simulink library "DEM_lib"  (Simulink 7.4)
settings: Solver=FixedStepDiscrete  StartTime=0.0  StopTime=Inf  FixedStep=0.001  RelTol=1e-3
undefined symbols (not defined in the file or in its folder): BCU_Drive_St, BCU_FastCharge_St, BCU_SlowCharge_St, COR_Fault_Bus, CTC_DefaultOffline_CtrCmd, CTC_DriveEmgyDcnct_CtrCmd, CTC_DriveOffline_CtrCmd, CTC_DriveOnline_CtrCmd, EHP_Fault_Bus, FCM_Fault_Bus, SCM_Fault_Bus
libraries: Defined_Functionality x82, simulink x2
(part 3 of 4)

== system DEM_lib/Diagnostic_Event_Management/fault_collect/BTM_Fault_Confirmed/Subsystem1 ==
  ifault : Inport  OutDataType=fixdt(1, 16)  OutScaling=2^0
  Terminator : Terminator
  Terminator1 : Terminator
  Terminator2 : Terminator
  diagnostic1 : Defined_Functionality/diagnostic1  SystemSampleTime=-1  afl_inc=DEMc_MdlTempOverfault_inc  afl_dec=DEMc_MdlTempOverfault_dec  afl_threshold=DEMc_MdlTempOverfault_AflThrld  aff_threshold=DEMc_MdlTempOverfault_AffThrld
      settings: AttributesFormatString=[AFL_INCREMENT=%<afl_inc>]\n[AFL_DECREMENT=%<afl_dec>]\n[AFL_THRESHOLD=%<afl_threshold>]\n[AFF_THRESHOLD=%<aff_threshold>]
  cfault : Outport  OutDataType=fixdt(1, 16)  OutScaling=2^0
  wires:
  ifault/1 -> diagnostic1/1
  diagnostic1/2 -> cfault/1
  diagnostic1/1 -> Terminator/1
  diagnostic1/4 -> Terminator1/1
  diagnostic1/3 -> Terminator2/1

== system DEM_lib/Diagnostic_Event_Management/fault_collect/BTM_Fault_Confirmed/Subsystem2 ==
  ifault : Inport  OutDataType=fixdt(1, 16)  OutScaling=2^0
  Terminator : Terminator
  Terminator1 : Terminator
  Terminator2 : Terminator
  diagnostic1 : Defined_Functionality/diagnostic1  SystemSampleTime=-1  afl_inc=DEMc_MdlTempOverwarn_inc  afl_dec=DEMc_MdlTempOverwarn_dec  afl_threshold=DEMc_MdlTempOverwarn_AflThrld  aff_threshold=DEMc_MdlTempOverwarn_AffThrld
      settings: AttributesFormatString=[AFL_INCREMENT=%<afl_inc>]\n[AFL_DECREMENT=%<afl_dec>]\n[AFL_THRESHOLD=%<afl_threshold>]\n[AFF_THRESHOLD=%<aff_threshold>]
  cfault : Outport  OutDataType=fixdt(1, 16)  OutScaling=2^0
  wires:
  diagnostic1/3 -> Terminator2/1
  diagnostic1/4 -> Terminator1/1
  diagnostic1/1 -> Terminator/1
  diagnostic1/2 -> cfault/1
  ifault/1 -> diagnostic1/1

== system DEM_lib/Diagnostic_Event_Management/fault_collect/BTM_Fault_Confirmed/Subsystem3 ==
  ifault : Inport  OutDataType=fixdt(1, 16)  OutScaling=2^0
  Terminator : Terminator
  Terminator1 : Terminator
  Terminator2 : Terminator
  diagnostic1 : Defined_Functionality/diagnostic1  SystemSampleTime=-1  afl_inc=DEMc_MdlTempUnderwarn_inc  afl_dec=DEMc_MdlTempUnderwarn_dec  afl_threshold=DEMc_MdlTempUnderwarn_AflThrld  aff_threshold=DEMc_MdlTempUnderwarn_AffThrld
      settings: AttributesFormatString=[AFL_INCREMENT=%<afl_inc>]\n[AFL_DECREMENT=%<afl_dec>]\n[AFL_THRESHOLD=%<afl_threshold>]\n[AFF_THRESHOLD=%<aff_threshold>]
  cfault : Outport  OutDataType=fixdt(1, 16)  OutScaling=2^0
  wires:
  diagnostic1/3 -> Terminator2/1
  diagnostic1/4 -> Terminator1/1
  diagnostic1/1 -> Terminator/1
  diagnostic1/2 -> cfault/1
  ifault/1 -> diagnostic1/1

== system DEM_lib/Diagnostic_Event_Management/fault_collect/BTM_Fault_Confirmed/Subsystem4 ==
  ifault : Inport  OutDataType=fixdt(1, 16)  OutScaling=2^0
  Terminator : Terminator
  Terminator1 : Terminator
  Terminator2 : Terminator
  diagnostic1 : Defined_Functionality/diagnostic1  SystemSampleTime=-1  afl_inc=DEMc_MdlTempDifOverwarn_inc  afl_dec=DEMc_MdlTempDifOverwarn_dec  afl_threshold=DEMc_MdlTempDifOverwarn_AflThrld  aff_threshold=DEMc_MdlTempDifOverwarn_AffThrld
      settings: AttributesFormatString=[AFL_INCREMENT=%<afl_inc>]\n[AFL_DECREMENT=%<afl_dec>]\n[AFL_THRESHOLD=%<afl_threshold>]\n[AFF_THRESHOLD=%<aff_threshold>]
  cfault : Outport  OutDataType=fixdt(1, 16)  OutScaling=2^0
  wires:
  ifault/1 -> diagnostic1/1
  diagnostic1/2 -> cfault/1
  diagnostic1/1 -> Terminator/1
  diagnostic1/4 -> Terminator1/1
  diagnostic1/3 -> Terminator2/1

== system DEM_lib/Diagnostic_Event_Management/fault_collect/BTM_Fault_Confirmed/Subsystem5 ==
  ifault : Inport  OutDataType=fixdt(1, 16)  OutScaling=2^0
  Terminator : Terminator
  Terminator1 : Terminator
  Terminator2 : Terminator
  diagnostic1 : Defined_Functionality/diagnostic1  SystemSampleTime=-1  afl_inc=DEMc_MdlTempDifOverfault_inc  afl_dec=DEMc_MdlTempDifOverfault_dec  afl_threshold=DEMc_MdlTempDifOverfault_AflThrld  aff_threshold=DEMc_MdlTempDifOverfault_AffThrld
      settings: AttributesFormatString=[AFL_INCREMENT=%<afl_inc>]\n[AFL_DECREMENT=%<afl_dec>]\n[AFL_THRESHOLD=%<afl_threshold>]\n[AFF_THRESHOLD=%<aff_threshold>]
  cfault : Outport  OutDataType=fixdt(1, 16)  OutScaling=2^0
  wires:
  diagnostic1/3 -> Terminator2/1
  diagnostic1/4 -> Terminator1/1
  diagnostic1/1 -> Terminator/1
  diagnostic1/2 -> cfault/1
  ifault/1 -> diagnostic1/1

== system DEM_lib/Diagnostic_Event_Management/fault_collect/BTM_Fault_Confirmed/Subsystem6 ==
  ifault : Inport  OutDataType=fixdt(1, 16)  OutScaling=2^0
  Terminator : Terminator
  Terminator1 : Terminator
  Terminator2 : Terminator
  diagnostic1 : Defined_Functionality/diagnostic1  SystemSampleTime=-1  afl_inc=DEMc_MdlTempOverfatal_inc  afl_dec=DEMc_MdlTempOverfatal_dec  afl_threshold=DEMc_MdlTempOverfatal_AflThrld  aff_threshold=DEMc_MdlTempOverfatal_AffThrld
      settings: AttributesFormatString=[AFL_INCREMENT=%<afl_inc>]\n[AFL_DECREMENT=%<afl_dec>]\n[AFL_THRESHOLD=%<afl_threshold>]\n[AFF_THRESHOLD=%<aff_threshold>]
  cfault : Outport  OutDataType=fixdt(1, 16)  OutScaling=2^0
  wires:
  diagnostic1/3 -> Terminator2/1
  diagnostic1/4 -> Terminator1/1
  diagnostic1/1 -> Terminator/1
  diagnostic1/2 -> cfault/1
  ifault/1 -> diagnostic1/1

== system DEM_lib/Diagnostic_Event_Management/fault_collect/BTM_Fault_Confirmed/Subsystem7 ==
  ifault : Inport  OutDataType=fixdt(1, 16)  OutScaling=2^0
  Terminator : Terminator
  Terminator1 : Terminator
  Terminator2 : Terminator
  diagnostic1 : Defined_Functionality/diagnostic1  SystemSampleTime=-1  afl_inc=DEMc_BMUMaxTempOverwarn_inc  afl_dec=DEMc_BMUMaxTempOverwarn_dec  afl_threshold=DEMc_BMUMaxTempOverwarn_AflThrld  aff_threshold=DEMc_BMUMaxTempOverwarn_AffThrld
      settings: AttributesFormatString=[AFL_INCREMENT=%<afl_inc>]\n[AFL_DECREMENT=%<afl_dec>]\n[AFL_THRESHOLD=%<afl_threshold>]\n[AFF_THRESHOLD=%<aff_threshold>]
  cfault : Outport  OutDataType=fixdt(1, 16)  OutScaling=2^0
  wires:
  ifault/1 -> diagnostic1/1
  diagnostic1/2 -> cfault/1
  diagnostic1/1 -> Terminator/1
  diagnostic1/4 -> Terminator1/1
  diagnostic1/3 -> Terminator2/1

== system DEM_lib/Diagnostic_Event_Management/fault_collect/BTM_Fault_Confirmed/Subsystem8 ==
  ifault : Inport  OutDataType=fixdt(1, 16)  OutScaling=2^0
  Terminator : Terminator
  Terminator1 : Terminator
  Terminator2 : Terminator
  diagnostic1 : Defined_Functionality/diagnostic1  SystemSampleTime=-1  afl_inc=DEMc_BCUMaxTempOverwarn_inc  afl_dec=DEMc_BCUMaxTempOverwarn_dec  afl_threshold=DEMc_BCUMaxTempOverwarn_AflThrld  aff_threshold=DEMc_BCUMaxTempOverwarn_AffThrld
      settings: AttributesFormatString=[AFL_INCREMENT=%<afl_inc>]\n[AFL_DECREMENT=%<afl_dec>]\n[AFL_THRESHOLD=%<afl_threshold>]\n[AFF_THRESHOLD=%<aff_threshold>]
  cfault : Outport  OutDataType=fixdt(1, 16)  OutScaling=2^0
  wires:
  diagnostic1/3 -> Terminator2/1
  diagnostic1/4 -> Terminator1/1
  diagnostic1/1 -> Terminator/1
  diagnostic1/2 -> cfault/1
  ifault/1 -> diagnostic1/1

== system DEM_lib/Diagnostic_Event_Management/fault_collect/COR_Fault_Confirmed/Subsystem1 ==
  ifault : Inport  OutDataType=fixdt(1, 16)  OutScaling=2^0
  Terminator : Terminator
  Terminator1 : Terminator
  Terminator2 : Terminator
  diagnostic1 : Defined_Functionality/diagnostic1  SystemSampleTime=-1  afl_inc=DEMc_CellCDcsefault_inc  afl_dec=DEMc_CellCDcsefault_dec  afl_threshold=DEMc_CellCDcsefault_AflThrld  aff_threshold=DEMc_CellCDcsefault_AffThrld
      settings: AttributesFormatString=[AFL_INCREMENT=%<afl_inc>]\n[AFL_DECREMENT=%<afl_dec>]\n[AFL_THRESHOLD=%<afl_threshold>]\n[AFF_THRESHOLD=%<aff_threshold>]
  cfault : Outport  OutDataType=fixdt(1, 16)  OutScaling=2^0
  wires:
  ifault/1 -> diagnostic1/1
  diagnostic1/2 -> cfault/1
  diagnostic1/1 -> Terminator/1
  diagnostic1/4 -> Terminator1/1
  diagnostic1/3 -> Terminator2/1

== system DEM_lib/Diagnostic_Event_Management/fault_collect/COR_Fault_Confirmed/Subsystem5 ==
  ifault : Inport  OutDataType=fixdt(1, 16)  OutScaling=2^0
  Terminator : Terminator
  Terminator1 : Terminator
  Terminator2 : Terminator
  diagnostic1 : Defined_Functionality/diagnostic1  SystemSampleTime=-1  afl_inc=DEMc_CellRDcsefault_inc  afl_dec=DEMc_CellRDcsefault_dec  afl_threshold=DEMc_CellRDcsefault_AflThrld  aff_threshold=DEMc_CellRDcsefault_AffThrld
      settings: AttributesFormatString=[AFL_INCREMENT=%<afl_inc>]\n[AFL_DECREMENT=%<afl_dec>]\n[AFL_THRESHOLD=%<afl_threshold>]\n[AFF_THRESHOLD=%<aff_threshold>]
  cfault : Outport  OutDataType=fixdt(1, 16)  OutScaling=2^0
  wires:
  diagnostic1/3 -> Terminator2/1
  diagnostic1/4 -> Terminator1/1
  diagnostic1/1 -> Terminator/1
  diagnostic1/2 -> cfault/1
  ifault/1 -> diagnostic1/1

== system DEM_lib/Diagnostic_Event_Management/fault_collect/COR_Fault_Confirmed/Subsystem8 ==
  ifault : Inport  OutDataType=fixdt(1, 16)  OutScaling=2^0
  Terminator : Terminator
  Terminator1 : Terminator
  Terminator2 : Terminator
  diagnostic1 : Defined_Functionality/diagnostic1  SystemSampleTime=-1  afl_inc=DEMc_CellRIcsefault_inc  afl_dec=DEMc_CellRIcsefault_dec  afl_threshold=DEMc_CellRIcsefault_AflThrld  aff_threshold=DEMc_CellRIcsefault_AffThrld
      settings: AttributesFormatString=[AFL_INCREMENT=%<afl_inc>]\n[AFL_DECREMENT=%<afl_dec>]\n[AFL_THRESHOLD=%<afl_threshold>]\n[AFF_THRESHOLD=%<aff_threshold>]
  cfault : Outport  OutDataType=fixdt(1, 16)  OutScaling=2^0
  wires:
  ifault/1 -> diagnostic1/1
  diagnostic1/2 -> cfault/1
  diagnostic1/1 -> Terminator/1
  diagnostic1/4 -> Terminator1/1
  diagnostic1/3 -> Terminator2/1

== system DEM_lib/Diagnostic_Event_Management/fault_collect/CTC_Fault_Confirmed/Subsystem1 ==
  ifault : Inport  OutDataType=fixdt(1, 16)  OutScaling=2^0
  Terminator : Terminator
  Terminator1 : Terminator
  Terminator2 : Terminator
  diagnostic1 : Defined_Functionality/diagnostic1  SystemSampleTime=-1  afl_inc=DEMc_PosCtrStuckOpenfault_inc  afl_dec=DEMc_PosCtrStuckOpenfault_dec  afl_threshold=DEMc_PosCtrStuckOpenfault_AflThrld  aff_threshold=DEMc_PosCtrStuckOpenfault_AffThrld
      settings: AttributesFormatString=[AFL_INCREMENT=%<afl_inc>]\n[AFL_DECREMENT=%<afl_dec>]\n[AFL_THRESHOLD=%<afl_threshold>]\n[AFF_THRESHOLD=%<aff_threshold>]
  cfault : Outport  OutDataType=fixdt(1, 16)  OutScaling=2^0
  wires:
  ifault/1 -> diagnostic1/1
  diagnostic1/2 -> cfault/1
  diagnostic1/1 -> Terminator/1
  diagnostic1/4 -> Terminator1/1
  diagnostic1/3 -> Terminator2/1

== system DEM_lib/Diagnostic_Event_Management/fault_collect/CTC_Fault_Confirmed/Subsystem10 ==
  ifault : Inport  OutDataType=fixdt(1, 16)  OutScaling=2^0
  Terminator : Terminator
  Terminator1 : Terminator
  Terminator2 : Terminator
  diagnostic1 : Defined_Functionality/diagnostic1  SystemSampleTime=-1  afl_inc=DEMc_HVEmcyDcnctTmOverfault_inc  afl_dec=DEMc_HVEmcyDcnctTmOverfault_dec  afl_threshold=DEMc_HVEmcyDcnctTmOverfault_AflThrld  aff_threshold=DEMc_HVEmcyDcnctTmOverfault_AffThrld
      settings: AttributesFormatString=[AFL_INCREMENT=%<afl_inc>]\n[AFL_DECREMENT=%<afl_dec>]\n[AFL_THRESHOLD=%<afl_threshold>]\n[AFF_THRESHOLD=%<aff_threshold>]
  cfault : Outport  OutDataType=fixdt(1, 16)  OutScaling=2^0
  wires:
  ifault/1 -> diagnostic1/1
  diagnostic1/2 -> cfault/1
  diagnostic1/1 -> Terminator/1
  diagnostic1/4 -> Terminator1/1
  diagnostic1/3 -> Terminator2/1

== system DEM_lib/Diagnostic_Event_Management/fault_collect/CTC_Fault_Confirmed/Subsystem11 ==
  ifault : Inport  OutDataType=fixdt(1, 16)  OutScaling=2^0
  Terminator : Terminator
  Terminator1 : Terminator
  Terminator2 : Terminator
  diagnostic1 : Defined_Functionality/diagnostic1  SystemSampleTime=-1  afl_inc=DEMc_PrecCurOverfault_inc  afl_dec=DEMc_PrecCurOverfault_dec  afl_threshold=DEMc_PrecCurOverfault_AflThrld  aff_threshold=DEMc_PrecCurOverfault_AffThrld
      settings: AttributesFormatString=[AFL_INCREMENT=%<afl_inc>]\n[AFL_DECREMENT=%<afl_dec>]\n[AFL_THRESHOLD=%<afl_threshold>]\n[AFF_THRESHOLD=%<aff_threshold>]
  cfault : Outport  OutDataType=fixdt(1, 16)  OutScaling=2^0
  wires:
  diagnostic1/3 -> Terminator2/1
  diagnostic1/4 -> Terminator1/1
  diagnostic1/1 -> Terminator/1
  diagnostic1/2 -> cfault/1
  ifault/1 -> diagnostic1/1

== system DEM_lib/Diagnostic_Event_Management/fault_collect/CTC_Fault_Confirmed/Subsystem12 ==
  ifault : Inport  OutDataType=fixdt(1, 16)  OutScaling=2^0
  Terminator : Terminator
  Terminator1 : Terminator
  Terminator2 : Terminator
  diagnostic1 : Defined_Functionality/diagnostic1  SystemSampleTime=-1  afl_inc=DEMc_HVCnctCurOverfault_inc  afl_dec=DEMc_HVCnctCurOverfault_dec  afl_threshold=DEMc_HVCnctCurOverfault_AflThrld  aff_threshold=DEMc_HVCnctCurOverfault_AffThrld
      settings: AttributesFormatString=[AFL_INCREMENT=%<afl_inc>]\n[AFL_DECREMENT=%<afl_dec>]\n[AFL_THRESHOLD=%<afl_threshold>]\n[AFF_THRESHOLD=%<aff_threshold>]
  cfault : Outport  OutDataType=fixdt(1, 16)  OutScaling=2^0
  wires:
  ifault/1 -> diagnostic1/1
  diagnostic1/2 -> cfault/1
  diagnostic1/1 -> Terminator/1
  diagnostic1/4 -> Terminator1/1
  diagnostic1/3 -> Terminator2/1

== system DEM_lib/Diagnostic_Event_Management/fault_collect/CTC_Fault_Confirmed/Subsystem3 ==
  ifault : Inport  OutDataType=fixdt(1, 16)  OutScaling=2^0
  Terminator : Terminator
  Terminator1 : Terminator
  Terminator2 : Terminator
  diagnostic1 : Defined_Functionality/diagnostic1  SystemSampleTime=-1  afl_inc=DEMc_PosCtrStuckCldfault_inc  afl_dec=DEMc_PosCtrStuckCldfault_dec  afl_threshold=DEMc_PosCtrStuckCldfault_AflThrld  aff_threshold=DEMc_PosCtrStuckCldfault_AffThrld
      settings: AttributesFormatString=[AFL_INCREMENT=%<afl_inc>]\n[AFL_DECREMENT=%<afl_dec>]\n[AFL_THRESHOLD=%<afl_threshold>]\n[AFF_THRESHOLD=%<aff_threshold>]
  cfault : Outport  OutDataType=fixdt(1, 16)  OutScaling=2^0
  wires:
  diagnostic1/3 -> Terminator2/1
  diagnostic1/4 -> Terminator1/1
  diagnostic1/1 -> Terminator/1
  diagnostic1/2 -> cfault/1
  ifault/1 -> diagnostic1/1

== system DEM_lib/Diagnostic_Event_Management/fault_collect/CTC_Fault_Confirmed/Subsystem4 ==
  ifault : Inport  OutDataType=fixdt(1, 16)  OutScaling=2^0
  Terminator : Terminator
  Terminator1 : Terminator
  Terminator2 : Terminator
  diagnostic1 : Defined_Functionality/diagnostic1  SystemSampleTime=-1  afl_inc=DEMc_NegCtrtStuckOpenfault_inc  afl_dec=DEMc_NegCtrtStuckOpenfault_dec  afl_threshold=DEMc_NegCtrtStuckOpenfault_AflThrld  aff_threshold=DEMc_NegCtrtStuckOpenfault_AffThrld
      settings: AttributesFormatString=[AFL_INCREMENT=%<afl_inc>]\n[AFL_DECREMENT=%<afl_dec>]\n[AFL_THRESHOLD=%<afl_threshold>]\n[AFF_THRESHOLD=%<aff_threshold>]
  cfault : Outport  OutDataType=fixdt(1, 16)  OutScaling=2^0
  wires:
  ifault/1 -> diagnostic1/1
  diagnostic1/2 -> cfault/1
  diagnostic1/1 -> Terminator/1
  diagnostic1/4 -> Terminator1/1
  diagnostic1/3 -> Terminator2/1

== system DEM_lib/Diagnostic_Event_Management/fault_collect/CTC_Fault_Confirmed/Subsystem5 ==
  ifault : Inport  OutDataType=fixdt(1, 16)  OutScaling=2^0
  Terminator : Terminator
  Terminator1 : Terminator
  Terminator2 : Terminator
  diagnostic1 : Defined_Functionality/diagnostic1  SystemSampleTime=-1  afl_inc=DEMc_NegCtrStuckCldfault_inc  afl_dec=DEMc_NegCtrStuckCldfault_dec  afl_threshold=DEMc_NegCtrStuckCldfault_AflThrld  aff_threshold=DEMc_NegCtrStuckCldfault_AffThrld
      settings: AttributesFormatString=[AFL_INCREMENT=%<afl_inc>]\n[AFL_DECREMENT=%<afl_dec>]\n[AFL_THRESHOLD=%<afl_threshold>]\n[AFF_THRESHOLD=%<aff_threshold>]
  cfault : Outport  OutDataType=fixdt(1, 16)  OutScaling=2^0
  wires:
  diagnostic1/3 -> Terminator2/1
  diagnostic1/4 -> Terminator1/1
  diagnostic1/1 -> Terminator/1
  diagnostic1/2 -> cfault/1
  ifault/1 -> diagnostic1/1

== system DEM_lib/Diagnostic_Event_Management/fault_collect/CTC_Fault_Confirmed/Subsystem6 ==
  ifault : Inport  OutDataType=fixdt(1, 16)  OutScaling=2^0
  Terminator : Terminator
  Terminator1 : Terminator
  Terminator2 : Terminator
  diagnostic1 : Defined_Functionality/diagnostic1  SystemSampleTime=-1  afl_inc=DEMc_PrecTmOverfault_inc  afl_dec=DEMc_PrecTmOverfault_dec  afl_threshold=DEMc_PrecTmOverfault_AflThrld  aff_threshold=DEMc_PrecTmOverfault_AffThrld
      settings: AttributesFormatString=[AFL_INCREMENT=%<afl_inc>]\n[AFL_DECREMENT=%<afl_dec>]\n[AFL_THRESHOLD=%<afl_threshold>]\n[AFF_THRESHOLD=%<aff_threshold>]
  cfault : Outport  OutDataType=fixdt(1, 16)  OutScaling=2^0
  wires:
  ifault/1 -> diagnostic1/1
  diagnostic1/2 -> cfault/1
  diagnostic1/1 -> Terminator/1
  diagnostic1/4 -> Terminator1/1
  diagnostic1/3 -> Terminator2/1

== system DEM_lib/Diagnostic_Event_Management/fault_collect/CTC_Fault_Confirmed/Subsystem7 ==
  ifault : Inport  OutDataType=fixdt(1, 16)  OutScaling=2^0
  Terminator : Terminator
  Terminator1 : Terminator
  Terminator2 : Terminator
  diagnostic1 : Defined_Functionality/diagnostic1  SystemSampleTime=-1  afl_inc=DEMc_HVCnctTmOverfault_inc  afl_dec=DEMc_HVCnctTmOverfault_dec  afl_threshold=DEMc_HVCnctTmOverfault_AflThrld  aff_threshold=DEMc_HVCnctTmOverfault_AffThrld
      settings: AttributesFormatString=[AFL_INCREMENT=%<afl_inc>]\n[AFL_DECREMENT=%<afl_dec>]\n[AFL_THRESHOLD=%<afl_threshold>]\n[AFF_THRESHOLD=%<aff_threshold>]
  cfault : Outport  OutDataType=fixdt(1, 16)  OutScaling=2^0
  wires:
  diagnostic1/3 -> Terminator2/1
  diagnostic1/4 -> Terminator1/1
  diagnostic1/1 -> Terminator/1
  diagnostic1/2 -> cfault/1
  ifault/1 -> diagnostic1/1

== system DEM_lib/Diagnostic_Event_Management/fault_collect/CTC_Fault_Confirmed/Subsystem8 ==
  ifault : Inport  OutDataType=fixdt(1, 16)  OutScaling=2^0
  Terminator : Terminator
  Terminator1 : Terminator
  Terminator2 : Terminator
  diagnostic1 : Defined_Functionality/diagnostic1  SystemSampleTime=-1  afl_inc=DEMc_HVDcncWaitTmOverfault_inc  afl_dec=DEMc_HVDcncWaitTmOverfault_dec  afl_threshold=DEMc_HVDcncWaitTmOverfault_AflThrld  aff_threshold=DEMc_HVDcncWaitTmOverfault_AffThrld
      settings: AttributesFormatString=[AFL_INCREMENT=%<afl_inc>]\n[AFL_DECREMENT=%<afl_dec>]\n[AFL_THRESHOLD=%<afl_threshold>]\n[AFF_THRESHOLD=%<aff_threshold>]
  cfault : Outport  OutDataType=fixdt(1, 16)  OutScaling=2^0
  wires:
  ifault/1 -> diagnostic1/1
  diagnostic1/2 -> cfault/1
  diagnostic1/1 -> Terminator/1
  diagnostic1/4 -> Terminator1/1
  diagnostic1/3 -> Terminator2/1

== system DEM_lib/Diagnostic_Event_Management/fault_collect/CTC_Fault_Confirmed/Subsystem9 ==
  ifault : Inport  OutDataType=fixdt(1, 16)  OutScaling=2^0
  Terminator : Terminator
  Terminator1 : Terminator
  Terminator2 : Terminator
  diagnostic1 : Defined_Functionality/diagnostic1  SystemSampleTime=-1  afl_inc=DEMc_HVDcnctTmOverfault_inc  afl_dec=DEMc_HVDcnctTmOverfault_dec  afl_threshold=DEMc_HVDcnctTmOverfault_AflThrld  aff_threshold=DEMc_HVDcnctTmOverfault_AffThrld
      settings: AttributesFormatString=[AFL_INCREMENT=%<afl_inc>]\n[AFL_DECREMENT=%<afl_dec>]\n[AFL_THRESHOLD=%<afl_threshold>]\n[AFF_THRESHOLD=%<aff_threshold>]
  cfault : Outport  OutDataType=fixdt(1, 16)  OutScaling=2^0
  wires:
  diagnostic1/3 -> Terminator2/1
  diagnostic1/4 -> Terminator1/1
  diagnostic1/1 -> Terminator/1
  diagnostic1/2 -> cfault/1
  ifault/1 -> diagnostic1/1

== system DEM_lib/Diagnostic_Event_Management/fault_collect/DefaultFaultBusAll/BAL ==
  Bus Creator1 : BusCreator  Inputs=1
  Constant36 : Constant  Value=0  OutDataTypeMode=boolean  OutDataType=fixdt(1, 16)  OutScaling=2^0  OutDataTypeStr=boolean
  BAL_Fault : Outport
  wires:
  Bus Creator1/1 -> BAL_Fault/1  "BAL_Fault_Bus"
  Constant36/1 -> Bus Creator1/1  "BALd_cflt_BalSwthAnml_warnRaw"

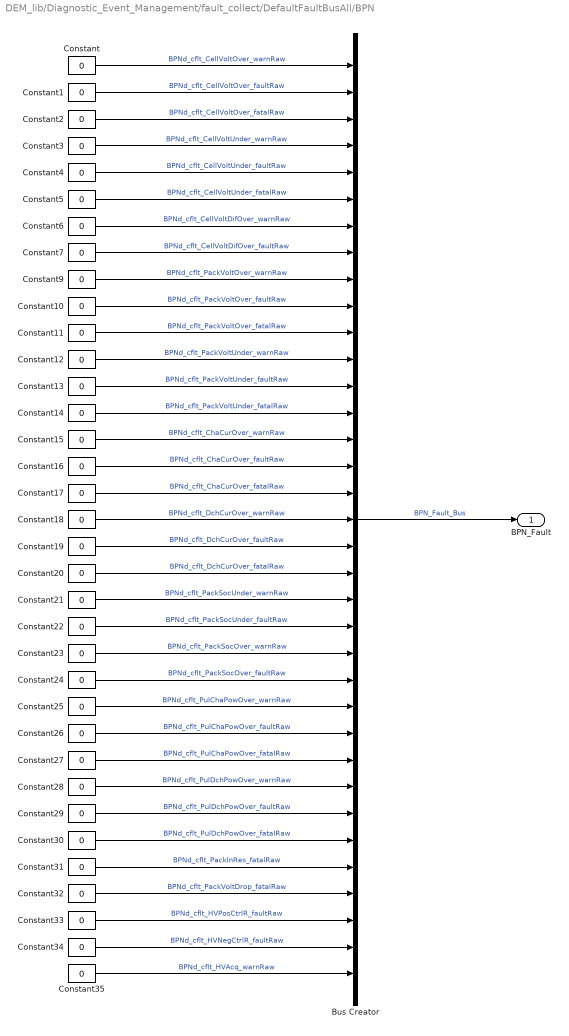
== system DEM_lib/Diagnostic_Event_Management/fault_collect/DefaultFaultBusAll/BPN ==
  Bus Creator : BusCreator  Inputs=35
  Constant{,1..7,9..35} (35 alike) : Constant  Value=0  OutDataTypeMode=boolean  OutDataType=fixdt(1, 16)  OutScaling=2^0  OutDataTypeStr=boolean
  BPN_Fault : Outport
  wires:
  Constant35/1 -> Bus Creator/35  "BPNd_cflt_HVAcq_warnRaw"
  Constant34/1 -> Bus Creator/34  "BPNd_cflt_HVNegCtrlR_faultRaw"
  Constant33/1 -> Bus Creator/33  "BPNd_cflt_HVPosCtrlR_faultRaw"
  Constant32/1 -> Bus Creator/32  "BPNd_cflt_PackVoltDrop_fatalRaw"
  Constant31/1 -> Bus Creator/31  "BPNd_cflt_PackInRes_fatalRaw"
  Constant30/1 -> Bus Creator/30  "BPNd_cflt_PulDchPowOver_fatalRaw"
  Constant29/1 -> Bus Creator/29  "BPNd_cflt_PulDchPowOver_faultRaw"
  Constant28/1 -> Bus Creator/28  "BPNd_cflt_PulDchPowOver_warnRaw"
  Constant27/1 -> Bus Creator/27  "BPNd_cflt_PulChaPowOver_fatalRaw"
  Constant26/1 -> Bus Creator/26  "BPNd_cflt_PulChaPowOver_faultRaw"
  Constant25/1 -> Bus Creator/25  "BPNd_cflt_PulChaPowOver_warnRaw"
  Constant24/1 -> Bus Creator/24  "BPNd_cflt_PackSocOver_faultRaw"
  Constant23/1 -> Bus Creator/23  "BPNd_cflt_PackSocOver_warnRaw"
  Constant22/1 -> Bus Creator/22  "BPNd_cflt_PackSocUnder_faultRaw"
  Constant21/1 -> Bus Creator/21  "BPNd_cflt_PackSocUnder_warnRaw"
  Constant20/1 -> Bus Creator/20  "BPNd_cflt_DchCurOver_fatalRaw"
  Constant19/1 -> Bus Creator/19  "BPNd_cflt_DchCurOver_faultRaw"
  Constant18/1 -> Bus Creator/18  "BPNd_cflt_DchCurOver_warnRaw"
  Constant17/1 -> Bus Creator/17  "BPNd_cflt_ChaCurOver_fatalRaw"
  Constant16/1 -> Bus Creator/16  "BPNd_cflt_ChaCurOver_faultRaw"
  Constant15/1 -> Bus Creator/15  "BPNd_cflt_ChaCurOver_warnRaw"
  Constant14/1 -> Bus Creator/14  "BPNd_cflt_PackVoltUnder_fatalRaw"
  Constant13/1 -> Bus Creator/13  "BPNd_cflt_PackVoltUnder_faultRaw"
  Constant12/1 -> Bus Creator/12  "BPNd_cflt_PackVoltUnder_warnRaw"
  Constant11/1 -> Bus Creator/11  "BPNd_cflt_PackVoltOver_fatalRaw"
  Constant10/1 -> Bus Creator/10  "BPNd_cflt_PackVoltOver_faultRaw"
  Constant9/1 -> Bus Creator/9  "BPNd_cflt_PackVoltOver_warnRaw"
  Bus Creator/1 -> BPN_Fault/1  "BPN_Fault_Bus"
  Constant7/1 -> Bus Creator/8  "BPNd_cflt_CellVoltDifOver_faultRaw"
  Constant6/1 -> Bus Creator/7  "BPNd_cflt_CellVoltDifOver_warnRaw"
  Constant5/1 -> Bus Creator/6  "BPNd_cflt_CellVoltUnder_fatalRaw"
  Constant4/1 -> Bus Creator/5  "BPNd_cflt_CellVoltUnder_faultRaw"
  Constant3/1 -> Bus Creator/4  "BPNd_cflt_CellVoltUnder_warnRaw"
  Constant2/1 -> Bus Creator/3  "BPNd_cflt_CellVoltOver_fatalRaw"
  Constant1/1 -> Bus Creator/2  "BPNd_cflt_CellVoltOver_faultRaw"
  Constant/1 -> Bus Creator/1  "BPNd_cflt_CellVoltOver_warnRaw"

== system DEM_lib/Diagnostic_Event_Management/fault_collect/DefaultFaultBusAll/BSC ==
  Bus Creator6 : BusCreator  Inputs=1
  Constant17 : Constant  Value=0  OutDataTypeMode=boolean  OutDataType=fixdt(1, 16)  OutScaling=2^0  OutDataTypeStr=boolean
  BSC_Fault : Outport
  wires:
  Bus Creator6/1 -> BSC_Fault/1  "BSC_Fault_Bus"
  Constant17/1 -> Bus Creator6/1  "BSCd_cflt_BCUFaultRaw"

== system DEM_lib/Diagnostic_Event_Management/fault_collect/DefaultFaultBusAll/BTM ==
  Bus Creator1 : BusCreator  Inputs=8
  Constant{6..8,36..40} (8 alike) : Constant  Value=0  OutDataTypeMode=boolean  OutDataType=fixdt(1, 16)  OutScaling=2^0  OutDataTypeStr=boolean
  BTM_Fault : Outport
  wires:
  Constant8/1 -> Bus Creator1/8  "BTMd_cflt_MdlTempDifOver_faultRaw"
  Constant7/1 -> Bus Creator1/7  "BTMd_cflt_MdlTempDifOver_warnRaw"
  Constant6/1 -> Bus Creator1/6  "BTMd_cflt_MdlTempUnder_warnRaw"
  Constant40/1 -> Bus Creator1/5  "BTMd_cflt_BCUMaxTempOver_warnRaw"
  Constant39/1 -> Bus Creator1/4  "BTMd_cflt_BMUMaxTempOver_warnRaw"
  Constant38/1 -> Bus Creator1/3  "BTMd_cflt_MdlTempOver_fatalRaw"
  Bus Creator1/1 -> BTM_Fault/1  "BTM_Fault_Bus"
  Constant37/1 -> Bus Creator1/2  "BTMd_cflt_MdlTempOver_faultRaw"
  Constant36/1 -> Bus Creator1/1  "BTMd_cflt_MdlTempOver_warnRaw"

== system DEM_lib/Diagnostic_Event_Management/fault_collect/DefaultFaultBusAll/COR ==
  Bus Creator1 : BusCreator  Inputs=3
  Constant37 : Constant  Value=0  OutDataTypeMode=boolean  OutDataType=fixdt(1, 16)  OutScaling=2^0  OutDataTypeStr=boolean
  Constant40 : Constant  Value=0  OutDataTypeMode=boolean  OutDataType=fixdt(1, 16)  OutScaling=2^0  OutDataTypeStr=boolean
  Constant43 : Constant  Value=0  OutDataTypeMode=boolean  OutDataType=fixdt(1, 16)  OutScaling=2^0  OutDataTypeStr=boolean
  COR_Fault : Outport
  wires:
  Constant43/1 -> Bus Creator1/3  "CORd_cflt_CellRIcse_faultRaw"
  Constant40/1 -> Bus Creator1/2  "CORd_cflt_CellRDcse_faultRaw"
  Constant37/1 -> Bus Creator1/1  "CORd_cflt_CellCDcse_faultRaw"
  Bus Creator1/1 -> COR_Fault/1  "COR_Fault_Bus"

== system DEM_lib/Diagnostic_Event_Management/fault_collect/DefaultFaultBusAll/CTC ==
  Bus Creator1 : BusCreator  Inputs=11
  Constant{15..25} (11 alike) : Constant  Value=0  OutDataTypeMode=boolean  OutDataType=fixdt(1, 16)  OutScaling=2^0  OutDataTypeStr=boolean
  CTC_Fault : Outport  OutDataType=fixdt(1, 16)  OutScaling=2^0
  wires:
  Constant17/1 -> Bus Creator1/11  "CTCd_cflt_HVCnctCurOver_faultRaw"
  Constant25/1 -> Bus Creator1/10  "CTCd_cflt_PrecCurOver_faultRaw"
  Constant24/1 -> Bus Creator1/9  "CTCd_cflt_HVEmcyDcnctTmOver_faultRaw"
  Constant23/1 -> Bus Creator1/8  "CTCd_cflt_HVDcnctTmOver_faultRaw"
  Constant22/1 -> Bus Creator1/7  "CTCd_cflt_HVDcncWaitTmOver_faultRaw"
  Constant21/1 -> Bus Creator1/6  "CTCd_cflt_HVCnctTmOver_faultRaw"
  Constant20/1 -> Bus Creator1/5  "CTCd_cflt_PrecTmOver_faultRaw"
  Constant19/1 -> Bus Creator1/4  "CTCd_cflt_NegCtrStuckCld_faultRaw"
  Constant18/1 -> Bus Creator1/3  "CTCd_cflt_NegCtrStuckOpen_faultRaw"
  Constant16/1 -> Bus Creator1/2  "CTCd_cflt_PosCtrStuckCld_faultRaw"
  Constant15/1 -> Bus Creator1/1  "CTCd_cflt_PosCtrStuckOpen_faultRaw"
  Bus Creator1/1 -> CTC_Fault/1  "CTC_Fault_Bus"

== system DEM_lib/Diagnostic_Event_Management/fault_collect/DefaultFaultBusAll/EHP ==
  Bus Creator1 : BusCreator  Inputs=5
  Constant{1..2,36..38} (5 alike) : Constant  Value=0  OutDataTypeMode=boolean  OutDataType=fixdt(1, 16)  OutScaling=2^0  OutDataTypeStr=boolean
  EHP_Fault : Outport
  wires:
  Constant2/1 -> Bus Creator1/5  "EHPd_cflt_HVILSt_faultRaw"
  Constant1/1 -> Bus Creator1/4  "EHPd_cflt_PosIso_warnRaw"
  Constant38/1 -> Bus Creator1/3  "EHPd_cflt_PosIso_faultRaw"
  Constant37/1 -> Bus Creator1/2  "EHPd_cflt_NegIso_warnRaw"
  Constant36/1 -> Bus Creator1/1  "EHPd_cflt_NegIso_faultRaw"
  Bus Creator1/1 -> EHP_Fault/1  "EHP_Fault_Bus"

== system DEM_lib/Diagnostic_Event_Management/fault_collect/DefaultFaultBusAll/FCM ==
  Bus Creator6 : BusCreator  Inputs=2
  Constant17 : Constant  Value=0  OutDataTypeMode=boolean  OutDataType=fixdt(1, 16)  OutScaling=2^0  OutDataTypeStr=boolean
  Constant18 : Constant  Value=0  OutDataTypeMode=boolean  OutDataType=fixdt(1, 16)  OutScaling=2^0  OutDataTypeStr=boolean
  FCM_Fault : Outport
  wires:
  Constant17/1 -> Bus Creator6/1  "FCMd_cflt_ChaCurDifOver_faultRaw"
  Constant18/1 -> Bus Creator6/2  "FCMd_cflt_ChaVoltDifOver_faultRaw"
  Bus Creator6/1 -> FCM_Fault/1  "FCM_Fault_Bus"

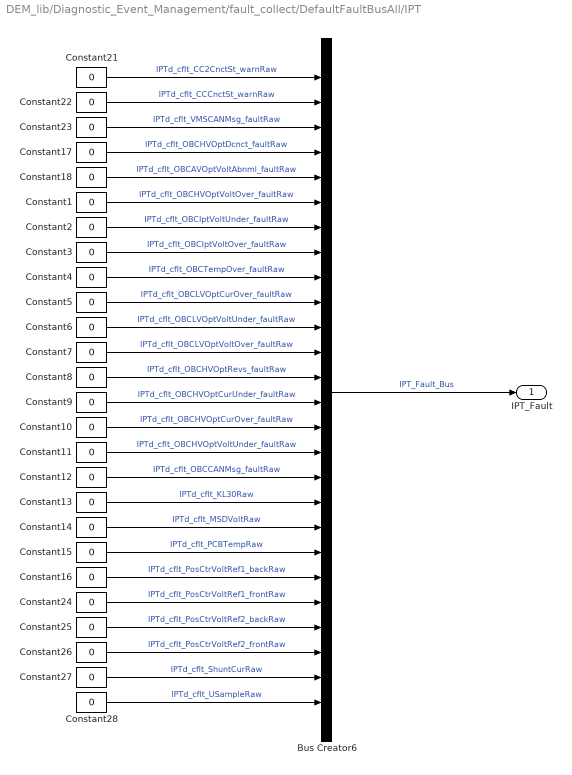
== system DEM_lib/Diagnostic_Event_Management/fault_collect/DefaultFaultBusAll/IPT ==
  Bus Creator6 : BusCreator  Inputs=26
  Constant{1..18,21..28} (26 alike) : Constant  Value=0  OutDataTypeMode=boolean  OutDataType=fixdt(1, 16)  OutScaling=2^0  OutDataTypeStr=boolean
  IPT_Fault : Outport
  wires:
  Constant18/1 -> Bus Creator6/5  "IPTd_cflt_OBCAVOptVoltAbnml_faultRaw"
  Constant17/1 -> Bus Creator6/4  "IPTd_cflt_OBCHVOptDcnct_faultRaw"
  Constant12/1 -> Bus Creator6/17  "IPTd_cflt_OBCCANMsg_faultRaw"
  Constant11/1 -> Bus Creator6/16  "IPTd_cflt_OBCHVOptVoltUnder_faultRaw"
  Constant10/1 -> Bus Creator6/15  "IPTd_cflt_OBCHVOptCurOver_faultRaw"
  Constant9/1 -> Bus Creator6/14  "IPTd_cflt_OBCHVOptCurUnder_faultRaw"
  Constant8/1 -> Bus Creator6/13  "IPTd_cflt_OBCHVOptRevs_faultRaw"
  Constant7/1 -> Bus Creator6/12  "IPTd_cflt_OBCLVOptVoltOver_faultRaw"
  Constant6/1 -> Bus Creator6/11  "IPTd_cflt_OBCLVOptVoltUnder_faultRaw"
  Constant5/1 -> Bus Creator6/10  "IPTd_cflt_OBCLVOptCurOver_faultRaw"
  Constant4/1 -> Bus Creator6/9  "IPTd_cflt_OBCTempOver_faultRaw"
  Constant3/1 -> Bus Creator6/8  "IPTd_cflt_OBCIptVoltOver_faultRaw"
  Constant2/1 -> Bus Creator6/7  "IPTd_cflt_OBCIptVoltUnder_faultRaw"
  Constant1/1 -> Bus Creator6/6  "IPTd_cflt_OBCHVOptVoltOver_faultRaw"
  Bus Creator6/1 -> IPT_Fault/1  "IPT_Fault_Bus"
  Constant23/1 -> Bus Creator6/3  "IPTd_cflt_VMSCANMsg_faultRaw"
  Constant22/1 -> Bus Creator6/2  "IPTd_cflt_CCCnctSt_warnRaw"
  Constant21/1 -> Bus Creator6/1  "IPTd_cflt_CC2CnctSt_warnRaw"
  Constant13/1 -> Bus Creator6/18  "IPTd_cflt_KL30Raw"
  Constant14/1 -> Bus Creator6/19  "IPTd_cflt_MSDVoltRaw"
  Constant15/1 -> Bus Creator6/20  "IPTd_cflt_PCBTempRaw"
  Constant16/1 -> Bus Creator6/21  "IPTd_cflt_PosCtrVoltRef1_backRaw"
  Constant24/1 -> Bus Creator6/22  "IPTd_cflt_PosCtrVoltRef1_frontRaw"
  Constant25/1 -> Bus Creator6/23  "IPTd_cflt_PosCtrVoltRef2_backRaw"
  Constant26/1 -> Bus Creator6/24  "IPTd_cflt_PosCtrVoltRef2_frontRaw"
  Constant27/1 -> Bus Creator6/25  "IPTd_cflt_ShuntCurRaw"
  Constant28/1 -> Bus Creator6/26  "IPTd_cflt_USampleRaw"

== system DEM_lib/Diagnostic_Event_Management/fault_collect/DefaultFaultBusAll/MCC ==
  Bus Creator6 : BusCreator  Inputs=1
  Constant17 : Constant  Value=0  OutDataTypeMode=boolean  OutDataType=fixdt(1, 16)  OutScaling=2^0  OutDataTypeStr=boolean
  MCC_Fault : Outport
  wires:
  Constant17/1 -> Bus Creator6/1  "MCCd_cflt_BMUInit_faultRaw"
  Bus Creator6/1 -> MCC_Fault/1  "MCC_Fault_Bus"

== system DEM_lib/Diagnostic_Event_Management/fault_collect/DefaultFaultBusAll/SCM ==
  Bus Creator6 : BusCreator  Inputs=2
  Constant17 : Constant  Value=0  OutDataTypeMode=boolean  OutDataType=fixdt(1, 16)  OutScaling=2^0  OutDataTypeStr=boolean
  Constant18 : Constant  Value=0  OutDataTypeMode=boolean  OutDataType=fixdt(1, 16)  OutScaling=2^0  OutDataTypeStr=boolean
  SCM_Fault : Outport
  wires:
  Constant17/1 -> Bus Creator6/1  "SCMd_cflt_CurOver_faultRaw"
  Constant18/1 -> Bus Creator6/2  "SCMd_cflt_VoltOver_faultRaw"
  Bus Creator6/1 -> SCM_Fault/1  "SCM_Fault_Bus"

== system DEM_lib/Diagnostic_Event_Management/fault_collect/EHP_Fault_Confirmed/Subsystem2 ==
  ifault : Inport  OutDataType=fixdt(1, 16)  OutScaling=2^0
  Terminator : Terminator
  Terminator1 : Terminator
  Terminator2 : Terminator
  diagnostic1 : Defined_Functionality/diagnostic1  SystemSampleTime=-1  afl_inc=DEMc_NegIsofault_inc  afl_dec=DEMc_NegIsofault_dec  afl_threshold=DEMc_NegIsofault_AflThrld  aff_threshold=DEMc_NegIsofault_AffThrld
      settings: AttributesFormatString=[AFL_INCREMENT=%<afl_inc>]\n[AFL_DECREMENT=%<afl_dec>]\n[AFL_THRESHOLD=%<afl_threshold>]\n[AFF_THRESHOLD=%<aff_threshold>]
  cfault : Outport  OutDataType=fixdt(1, 16)  OutScaling=2^0
  wires:
  diagnostic1/3 -> Terminator2/1
  diagnostic1/4 -> Terminator1/1
  diagnostic1/1 -> Terminator/1
  diagnostic1/2 -> cfault/1
  ifault/1 -> diagnostic1/1

== system DEM_lib/Diagnostic_Event_Management/fault_collect/EHP_Fault_Confirmed/Subsystem4 ==
  ifault : Inport  OutDataType=fixdt(1, 16)  OutScaling=2^0
  Terminator : Terminator
  Terminator1 : Terminator
  Terminator2 : Terminator
  diagnostic1 : Defined_Functionality/diagnostic1  SystemSampleTime=-1  afl_inc=DEMc_NegIsowarn_inc  afl_dec=DEMc_NegIsowarn_dec  afl_threshold=DEMc_NegIsowarn_AflThrld  aff_threshold=DEMc_NegIsowarn_AffThrld
      settings: AttributesFormatString=[AFL_INCREMENT=%<afl_inc>]\n[AFL_DECREMENT=%<afl_dec>]\n[AFL_THRESHOLD=%<afl_threshold>]\n[AFF_THRESHOLD=%<aff_threshold>]
  cfault : Outport  OutDataType=fixdt(1, 16)  OutScaling=2^0
  wires:
  ifault/1 -> diagnostic1/1
  diagnostic1/2 -> cfault/1
  diagnostic1/1 -> Terminator/1
  diagnostic1/4 -> Terminator1/1
  diagnostic1/3 -> Terminator2/1

== system DEM_lib/Diagnostic_Event_Management/fault_collect/EHP_Fault_Confirmed/Subsystem5 ==
  ifault : Inport  OutDataType=fixdt(1, 16)  OutScaling=2^0
  Terminator : Terminator
  Terminator1 : Terminator
  Terminator2 : Terminator
  diagnostic1 : Defined_Functionality/diagnostic1  SystemSampleTime=-1  afl_inc=DEMc_PosIsofault_inc  afl_dec=DEMc_PosIsofault_dec  afl_threshold=DEMc_PosIsofault_AflThrld  aff_threshold=DEMc_PosIsofault_AffThrld
      settings: AttributesFormatString=[AFL_INCREMENT=%<afl_inc>]\n[AFL_DECREMENT=%<afl_dec>]\n[AFL_THRESHOLD=%<afl_threshold>]\n[AFF_THRESHOLD=%<aff_threshold>]
  cfault : Outport  OutDataType=fixdt(1, 16)  OutScaling=2^0
  wires:
  diagnostic1/3 -> Terminator2/1
  diagnostic1/4 -> Terminator1/1
  diagnostic1/1 -> Terminator/1
  diagnostic1/2 -> cfault/1
  ifault/1 -> diagnostic1/1

== system DEM_lib/Diagnostic_Event_Management/fault_collect/EHP_Fault_Confirmed/Subsystem6 ==
  ifault : Inport  OutDataType=fixdt(1, 16)  OutScaling=2^0
  Terminator : Terminator
  Terminator1 : Terminator
  Terminator2 : Terminator
  diagnostic1 : Defined_Functionality/diagnostic1  SystemSampleTime=-1  afl_inc=DEMc_PosIsowarn_inc  afl_dec=DEMc_PosIsowarn_dec  afl_threshold=DEMc_PosIsowarn_AflThrld  aff_threshold=DEMc_PosIsowarn_AffThrld
      settings: AttributesFormatString=[AFL_INCREMENT=%<afl_inc>]\n[AFL_DECREMENT=%<afl_dec>]\n[AFL_THRESHOLD=%<afl_threshold>]\n[AFF_THRESHOLD=%<aff_threshold>]
  cfault : Outport  OutDataType=fixdt(1, 16)  OutScaling=2^0
  wires:
  ifault/1 -> diagnostic1/1
  diagnostic1/2 -> cfault/1
  diagnostic1/1 -> Terminator/1
  diagnostic1/4 -> Terminator1/1
  diagnostic1/3 -> Terminator2/1

== system DEM_lib/Diagnostic_Event_Management/fault_collect/EHP_Fault_Confirmed/Subsystem7 ==
  ifault : Inport  OutDataType=fixdt(1, 16)  OutScaling=2^0
  Terminator : Terminator
  Terminator1 : Terminator
  Terminator2 : Terminator
  diagnostic1 : Defined_Functionality/diagnostic1  SystemSampleTime=-1  afl_inc=DEMc_HVILSt_inc  afl_dec=DEMc_HVILSt_dec  afl_threshold=DEMc_HVILSt_AflThrld  aff_threshold=DEMc_HVILSt_AffThrld
      settings: AttributesFormatString=[AFL_INCREMENT=%<afl_inc>]\n[AFL_DECREMENT=%<afl_dec>]\n[AFL_THRESHOLD=%<afl_threshold>]\n[AFF_THRESHOLD=%<aff_threshold>]
  cfault : Outport  OutDataType=fixdt(1, 16)  OutScaling=2^0
  wires:
  diagnostic1/3 -> Terminator2/1
  diagnostic1/4 -> Terminator1/1
  diagnostic1/1 -> Terminator/1
  diagnostic1/2 -> cfault/1
  ifault/1 -> diagnostic1/1

== system DEM_lib/Diagnostic_Event_Management/fault_collect/FCM_Fault_Confirmed/Subsystem1 ==
  ifault : Inport  OutDataType=fixdt(1, 16)  OutScaling=2^0
  Terminator : Terminator
  Terminator1 : Terminator
  Terminator2 : Terminator
  diagnostic1 : Defined_Functionality/diagnostic1  SystemSampleTime=-1  afl_inc=1  afl_dec=2  afl_threshold=10  aff_threshold=255
      settings: AttributesFormatString=[AFL_INCREMENT=%<afl_inc>]\n[AFL_DECREMENT=%<afl_dec>]\n[AFL_THRESHOLD=%<afl_threshold>]\n[AFF_THRESHOLD=%<aff_threshold>]
  cfault : Outport  OutDataType=fixdt(1, 16)  OutScaling=2^0
  wires:
  ifault/1 -> diagnostic1/1
  diagnostic1/2 -> cfault/1
  diagnostic1/1 -> Terminator/1
  diagnostic1/4 -> Terminator1/1
  diagnostic1/3 -> Terminator2/1

== system DEM_lib/Diagnostic_Event_Management/fault_collect/FCM_Fault_Confirmed/Subsystem2 ==
  ifault : Inport  OutDataType=fixdt(1, 16)  OutScaling=2^0
  Terminator : Terminator
  Terminator1 : Terminator
  Terminator2 : Terminator
  diagnostic1 : Defined_Functionality/diagnostic1  SystemSampleTime=-1  afl_inc=1  afl_dec=2  afl_threshold=10  aff_threshold=255
      settings: AttributesFormatString=[AFL_INCREMENT=%<afl_inc>]\n[AFL_DECREMENT=%<afl_dec>]\n[AFL_THRESHOLD=%<afl_threshold>]\n[AFF_THRESHOLD=%<aff_threshold>]
  cfault : Outport  OutDataType=fixdt(1, 16)  OutScaling=2^0
  wires:
  diagnostic1/3 -> Terminator2/1
  diagnostic1/4 -> Terminator1/1
  diagnostic1/1 -> Terminator/1
  diagnostic1/2 -> cfault/1
  ifault/1 -> diagnostic1/1

== system DEM_lib/Diagnostic_Event_Management/fault_collect/IPT_Fault_Confirmed/Subsystem20 ==
  ifault : Inport  OutDataType=fixdt(1, 16)  OutScaling=2^0
  Terminator : Terminator
  Terminator1 : Terminator
  Terminator2 : Terminator
  diagnostic1 : Defined_Functionality/diagnostic1  SystemSampleTime=-1  afl_inc=1  afl_dec=2  afl_threshold=10  aff_threshold=255
      settings: AttributesFormatString=[AFL_INCREMENT=%<afl_inc>]\n[AFL_DECREMENT=%<afl_dec>]\n[AFL_THRESHOLD=%<afl_threshold>]\n[AFF_THRESHOLD=%<aff_threshold>]
  cfault : Outport  OutDataType=fixdt(1, 16)  OutScaling=2^0
  wires:
  diagnostic1/3 -> Terminator2/1
  diagnostic1/4 -> Terminator1/1
  diagnostic1/1 -> Terminator/1
  diagnostic1/2 -> cfault/1
  ifault/1 -> diagnostic1/1

== system DEM_lib/Diagnostic_Event_Management/fault_collect/IPT_Fault_Confirmed/Subsystem21 ==
  ifault : Inport  OutDataType=fixdt(1, 16)  OutScaling=2^0
  Terminator : Terminator
  Terminator1 : Terminator
  Terminator2 : Terminator
  diagnostic1 : Defined_Functionality/diagnostic1  SystemSampleTime=-1  afl_inc=1  afl_dec=2  afl_threshold=10  aff_threshold=255
      settings: AttributesFormatString=[AFL_INCREMENT=%<afl_inc>]\n[AFL_DECREMENT=%<afl_dec>]\n[AFL_THRESHOLD=%<afl_threshold>]\n[AFF_THRESHOLD=%<aff_threshold>]
  cfault : Outport  OutDataType=fixdt(1, 16)  OutScaling=2^0
  wires:
  diagnostic1/3 -> Terminator2/1
  diagnostic1/4 -> Terminator1/1
  diagnostic1/1 -> Terminator/1
  diagnostic1/2 -> cfault/1
  ifault/1 -> diagnostic1/1

== system DEM_lib/Diagnostic_Event_Management/fault_collect/IPT_Fault_Confirmed/Subsystem22 ==
  ifault : Inport  OutDataType=fixdt(1, 16)  OutScaling=2^0
  Terminator : Terminator
  Terminator1 : Terminator
  Terminator2 : Terminator
  diagnostic1 : Defined_Functionality/diagnostic1  SystemSampleTime=-1  afl_inc=1  afl_dec=2  afl_threshold=10  aff_threshold=255
      settings: AttributesFormatString=[AFL_INCREMENT=%<afl_inc>]\n[AFL_DECREMENT=%<afl_dec>]\n[AFL_THRESHOLD=%<afl_threshold>]\n[AFF_THRESHOLD=%<aff_threshold>]
  cfault : Outport  OutDataType=fixdt(1, 16)  OutScaling=2^0
  wires:
  ifault/1 -> diagnostic1/1
  diagnostic1/2 -> cfault/1
  diagnostic1/1 -> Terminator/1
  diagnostic1/4 -> Terminator1/1
  diagnostic1/3 -> Terminator2/1

== system DEM_lib/Diagnostic_Event_Management/fault_collect/IPT_Fault_Confirmed/Subsystem23 ==
  ifault : Inport  OutDataType=fixdt(1, 16)  OutScaling=2^0
  Terminator : Terminator
  Terminator1 : Terminator
  Terminator2 : Terminator
  diagnostic1 : Defined_Functionality/diagnostic1  SystemSampleTime=-1  afl_inc=1  afl_dec=2  afl_threshold=10  aff_threshold=255
      settings: AttributesFormatString=[AFL_INCREMENT=%<afl_inc>]\n[AFL_DECREMENT=%<afl_dec>]\n[AFL_THRESHOLD=%<afl_threshold>]\n[AFF_THRESHOLD=%<aff_threshold>]
  cfault : Outport  OutDataType=fixdt(1, 16)  OutScaling=2^0
  wires:
  ifault/1 -> diagnostic1/1
  diagnostic1/2 -> cfault/1
  diagnostic1/1 -> Terminator/1
  diagnostic1/4 -> Terminator1/1
  diagnostic1/3 -> Terminator2/1

== system DEM_lib/Diagnostic_Event_Management/fault_collect/IPT_Fault_Confirmed/Subsystem24 ==
  ifault : Inport  OutDataType=fixdt(1, 16)  OutScaling=2^0
  Terminator : Terminator
  Terminator1 : Terminator
  Terminator2 : Terminator
  diagnostic1 : Defined_Functionality/diagnostic1  SystemSampleTime=-1  afl_inc=1  afl_dec=2  afl_threshold=10  aff_threshold=255
      settings: AttributesFormatString=[AFL_INCREMENT=%<afl_inc>]\n[AFL_DECREMENT=%<afl_dec>]\n[AFL_THRESHOLD=%<afl_threshold>]\n[AFF_THRESHOLD=%<aff_threshold>]
  cfault : Outport  OutDataType=fixdt(1, 16)  OutScaling=2^0
  wires:
  diagnostic1/3 -> Terminator2/1
  diagnostic1/4 -> Terminator1/1
  diagnostic1/1 -> Terminator/1
  diagnostic1/2 -> cfault/1
  ifault/1 -> diagnostic1/1

== system DEM_lib/Diagnostic_Event_Management/fault_collect/IPT_Fault_Confirmed/Subsystem25 ==
  ifault : Inport  OutDataType=fixdt(1, 16)  OutScaling=2^0
  Terminator : Terminator
  Terminator1 : Terminator
  Terminator2 : Terminator
  diagnostic1 : Defined_Functionality/diagnostic1  SystemSampleTime=-1  afl_inc=1  afl_dec=2  afl_threshold=10  aff_threshold=255
      settings: AttributesFormatString=[AFL_INCREMENT=%<afl_inc>]\n[AFL_DECREMENT=%<afl_dec>]\n[AFL_THRESHOLD=%<afl_threshold>]\n[AFF_THRESHOLD=%<aff_threshold>]
  cfault : Outport  OutDataType=fixdt(1, 16)  OutScaling=2^0
  wires:
  ifault/1 -> diagnostic1/1
  diagnostic1/2 -> cfault/1
  diagnostic1/1 -> Terminator/1
  diagnostic1/4 -> Terminator1/1
  diagnostic1/3 -> Terminator2/1

== system DEM_lib/Diagnostic_Event_Management/fault_collect/IPT_Fault_Confirmed/Subsystem26 ==
  ifault : Inport  OutDataType=fixdt(1, 16)  OutScaling=2^0
  Terminator : Terminator
  Terminator1 : Terminator
  Terminator2 : Terminator
  diagnostic1 : Defined_Functionality/diagnostic1  SystemSampleTime=-1  afl_inc=1  afl_dec=2  afl_threshold=10  aff_threshold=255
      settings: AttributesFormatString=[AFL_INCREMENT=%<afl_inc>]\n[AFL_DECREMENT=%<afl_dec>]\n[AFL_THRESHOLD=%<afl_threshold>]\n[AFF_THRESHOLD=%<aff_threshold>]
  cfault : Outport  OutDataType=fixdt(1, 16)  OutScaling=2^0
  wires:
  diagnostic1/3 -> Terminator2/1
  diagnostic1/4 -> Terminator1/1
  diagnostic1/1 -> Terminator/1
  diagnostic1/2 -> cfault/1
  ifault/1 -> diagnostic1/1

== system DEM_lib/Diagnostic_Event_Management/fault_collect/IPT_Fault_Confirmed/Subsystem27 ==
  ifault : Inport  OutDataType=fixdt(1, 16)  OutScaling=2^0
  Terminator : Terminator
  Terminator1 : Terminator
  Terminator2 : Terminator
  diagnostic1 : Defined_Functionality/diagnostic1  SystemSampleTime=-1  afl_inc=1  afl_dec=2  afl_threshold=10  aff_threshold=255
      settings: AttributesFormatString=[AFL_INCREMENT=%<afl_inc>]\n[AFL_DECREMENT=%<afl_dec>]\n[AFL_THRESHOLD=%<afl_threshold>]\n[AFF_THRESHOLD=%<aff_threshold>]
  cfault : Outport  OutDataType=fixdt(1, 16)  OutScaling=2^0
  wires:
  diagnostic1/3 -> Terminator2/1
  diagnostic1/4 -> Terminator1/1
  diagnostic1/1 -> Terminator/1
  diagnostic1/2 -> cfault/1
  ifault/1 -> diagnostic1/1

== system DEM_lib/Diagnostic_Event_Management/fault_collect/IPT_Fault_Confirmed/Subsystem28 ==
  ifault : Inport  OutDataType=fixdt(1, 16)  OutScaling=2^0
  Terminator : Terminator
  Terminator1 : Terminator
  Terminator2 : Terminator
  diagnostic1 : Defined_Functionality/diagnostic1  SystemSampleTime=-1  afl_inc=1  afl_dec=2  afl_threshold=10  aff_threshold=255
      settings: AttributesFormatString=[AFL_INCREMENT=%<afl_inc>]\n[AFL_DECREMENT=%<afl_dec>]\n[AFL_THRESHOLD=%<afl_threshold>]\n[AFF_THRESHOLD=%<aff_threshold>]
  cfault : Outport  OutDataType=fixdt(1, 16)  OutScaling=2^0
  wires:
  ifault/1 -> diagnostic1/1
  diagnostic1/2 -> cfault/1
  diagnostic1/1 -> Terminator/1
  diagnostic1/4 -> Terminator1/1
  diagnostic1/3 -> Terminator2/1

== system DEM_lib/Diagnostic_Event_Management/fault_collect/IPT_Fault_Confirmed/Subsystem5 ==
  ifault : Inport  OutDataType=fixdt(1, 16)  OutScaling=2^0
  Terminator : Terminator
  Terminator1 : Terminator
  Terminator2 : Terminator
  diagnostic1 : Defined_Functionality/diagnostic1  SystemSampleTime=-1  afl_inc=DEMc_CC2CnctStwarn_inc  afl_dec=DEMc_CC2CnctStwarn_dec  afl_threshold=DEMc_CC2CnctStwarn_AflThrld  aff_threshold=DEMc_CC2CnctStwarn_AffThrld
      settings: AttributesFormatString=[AFL_INCREMENT=%<afl_inc>]\n[AFL_DECREMENT=%<afl_dec>]\n[AFL_THRESHOLD=%<afl_threshold>]\n[AFF_THRESHOLD=%<aff_threshold>]
  cfault : Outport  OutDataType=fixdt(1, 16)  OutScaling=2^0
  wires:
  diagnostic1/3 -> Terminator2/1
  diagnostic1/4 -> Terminator1/1
  diagnostic1/1 -> Terminator/1
  diagnostic1/2 -> cfault/1
  ifault/1 -> diagnostic1/1

== system DEM_lib/Diagnostic_Event_Management/fault_collect/IPT_Fault_Confirmed/Subsystem6 ==
  ifault : Inport  OutDataType=fixdt(1, 16)  OutScaling=2^0
  Terminator : Terminator
  Terminator1 : Terminator
  Terminator2 : Terminator
  diagnostic1 : Defined_Functionality/diagnostic1  SystemSampleTime=-1  afl_inc=DEMc_CCCnctStwarn_inc  afl_dec=DEMc_CCCnctStwarn_dec  afl_threshold=DEMc_CCCnctStwarn_AflThrld  aff_threshold=DEMc_CCCnctStwarn_AffThrld
      settings: AttributesFormatString=[AFL_INCREMENT=%<afl_inc>]\n[AFL_DECREMENT=%<afl_dec>]\n[AFL_THRESHOLD=%<afl_threshold>]\n[AFF_THRESHOLD=%<aff_threshold>]
  cfault : Outport  OutDataType=fixdt(1, 16)  OutScaling=2^0
  wires:
  ifault/1 -> diagnostic1/1
  diagnostic1/2 -> cfault/1
  diagnostic1/1 -> Terminator/1
  diagnostic1/4 -> Terminator1/1
  diagnostic1/3 -> Terminator2/1

== system DEM_lib/Diagnostic_Event_Management/fault_collect/IPT_Fault_Confirmed/Subsystem7 ==
  ifault : Inport  OutDataType=fixdt(1, 16)  OutScaling=2^0
  Terminator : Terminator
  Terminator1 : Terminator
  Terminator2 : Terminator
  diagnostic1 : Defined_Functionality/diagnostic1  SystemSampleTime=-1  afl_inc=DEMc_CANMsgfault_inc  afl_dec=DEMc_CANMsgfault_dec  afl_threshold=DEMc_CANMsgfault_AflThrld  aff_threshold=DEMc_CANMsgfault_AffThrld
      settings: AttributesFormatString=[AFL_INCREMENT=%<afl_inc>]\n[AFL_DECREMENT=%<afl_dec>]\n[AFL_THRESHOLD=%<afl_threshold>]\n[AFF_THRESHOLD=%<aff_threshold>]
  cfault : Outport  OutDataType=fixdt(1, 16)  OutScaling=2^0
  wires:
  diagnostic1/3 -> Terminator2/1
  diagnostic1/4 -> Terminator1/1
  diagnostic1/1 -> Terminator/1
  diagnostic1/2 -> cfault/1
  ifault/1 -> diagnostic1/1

== system DEM_lib/Diagnostic_Event_Management/fault_collect/MCC_Fault_Confirmed/Subsystem2 ==
  ifault : Inport  OutDataType=fixdt(1, 16)  OutScaling=2^0
  Terminator : Terminator
  Terminator1 : Terminator
  Terminator2 : Terminator
  diagnostic1 : Defined_Functionality/diagnostic1  SystemSampleTime=-1  afl_inc=1  afl_dec=2  afl_threshold=10  aff_threshold=255
      settings: AttributesFormatString=[AFL_INCREMENT=%<afl_inc>]\n[AFL_DECREMENT=%<afl_dec>]\n[AFL_THRESHOLD=%<afl_threshold>]\n[AFF_THRESHOLD=%<aff_threshold>]
  cfault : Outport  OutDataType=fixdt(1, 16)  OutScaling=2^0
  wires:
  ifault/1 -> diagnostic1/1
  diagnostic1/2 -> cfault/1
  diagnostic1/1 -> Terminator/1
  diagnostic1/4 -> Terminator1/1
  diagnostic1/3 -> Terminator2/1

== system DEM_lib/Diagnostic_Event_Management/fault_collect/SCM_Fault_Confirmed/Subsystem1 ==
  ifault : Inport  OutDataType=fixdt(1, 16)  OutScaling=2^0
  Terminator : Terminator
  Terminator1 : Terminator
  Terminator2 : Terminator
  diagnostic1 : Defined_Functionality/diagnostic1  SystemSampleTime=-1  afl_inc=1  afl_dec=2  afl_threshold=10  aff_threshold=255
      settings: AttributesFormatString=[AFL_INCREMENT=%<afl_inc>]\n[AFL_DECREMENT=%<afl_dec>]\n[AFL_THRESHOLD=%<afl_threshold>]\n[AFF_THRESHOLD=%<aff_threshold>]
  cfault : Outport  OutDataType=fixdt(1, 16)  OutScaling=2^0
  wires:
  diagnostic1/3 -> Terminator2/1
  diagnostic1/4 -> Terminator1/1
  diagnostic1/1 -> Terminator/1
  diagnostic1/2 -> cfault/1
  ifault/1 -> diagnostic1/1

== system DEM_lib/Diagnostic_Event_Management/fault_collect/SCM_Fault_Confirmed/Subsystem2 ==
  ifault : Inport  OutDataType=fixdt(1, 16)  OutScaling=2^0
  Terminator : Terminator
  Terminator1 : Terminator
  Terminator2 : Terminator
  diagnostic1 : Defined_Functionality/diagnostic1  SystemSampleTime=-1  afl_inc=1  afl_dec=2  afl_threshold=10  aff_threshold=255
      settings: AttributesFormatString=[AFL_INCREMENT=%<afl_inc>]\n[AFL_DECREMENT=%<afl_dec>]\n[AFL_THRESHOLD=%<afl_threshold>]\n[AFF_THRESHOLD=%<aff_threshold>]
  cfault : Outport  OutDataType=fixdt(1, 16)  OutScaling=2^0
  wires:
  ifault/1 -> diagnostic1/1
  diagnostic1/2 -> cfault/1
  diagnostic1/1 -> Terminator/1
  diagnostic1/4 -> Terminator1/1
  diagnostic1/3 -> Terminator2/1
